simulink model "F103_0804_simulink_model"  (R2025b)
settings: Solver=FixedStepDiscrete  StartTime=0.0  StopTime=10.0  FixedStep=0.01  RelTol=1e-3  EnableMultiTasking=on
settings Model: Creator=Admin1  LastModifiedBy=Admin1
settings SolverCC: AutoInsertRateTranBlk=on
settings OptimizationCC: DefaultParameterBehavior=Inlined  UseDivisionForNetSlopeComputation=on  GainParamInheritBuiltInType=on  UseFloatMulNetSlope=on  InlineInvariantSignals=on  PassReuseOutputArgsAs=Individual arguments  ZeroExternalMemoryAtStartup=off  ZeroInternalMemoryAtStartup=off  NoFixptDivByZeroProtection=on  EfficientFloat2IntCast=on  LifeSpan=1  OptimizeBlockOrder=speed  DifferentSizesBufferReuse=on  EfficientTunableParamExpr=on
settings DebuggingCC: ParameterTunabilityLossMsg=error
settings HardwareCC: ProdBitPerPointer=32.0  ProdBitPerSizeT=32.0  ProdBitPerPtrDiffT=32.0  ProdLargestAtomicInteger=Long  ProdLargestAtomicFloat=Double  ProdWordSize=32.0  ProdLongLongMode=on  ProdHWDeviceType=ARM Compatible->STM32Processor
settings SFSimCC: SimCustomHeaderCode=bms_app.h  SimUserSources=bms_app.c  SimUserIncludeDirs=D:\FSAE_CHD\BMS\STM32_LTC68xx_BMS_Chang-an\F407_VET6_Test\Appl  MATLABDynamicMemAlloc=off
settings RTWCC: SystemTargetFile=ert.tlc  GenCodeOnly=on  TemplateMakefile=ert_default_tmf  CustomHeaderCode=bms_app.h  CustomInclude=D:\FSAE_CHD\BMS\STM32_LTC68xx_BMS_Chang-an\F407_VET6_Test\Appl  CustomSource=bms_app.c  Description=Embedded Coder
settings CodeAppCC: ForceParamTrailComments=on  IgnoreCustomStorageClasses=off  OperatorAnnotations=on  SimulinkDataObjDesc=on  SFDataObjDesc=on  CustomSymbolStrGlobalVar=rt$N$M  CustomSymbolStrType=$N$M  CustomSymbolStrFcn=$N$M$F  CustomSymbolStrMacro=$N$M  InsertBlockDesc=on
settings ERTTargetCC: ERTCustomFileTemplate=example_file_process.tlc  ERTFilePackagingFormat=CompactWithDataFile  TargetLangStandard=C99 (ISO)  IncludeMdlTerminateFcn=off  CombineSignalStateStructs=on  SupportAbsoluteTime=off  SupportComplex=off  SupportNonInlinedSFcns=on

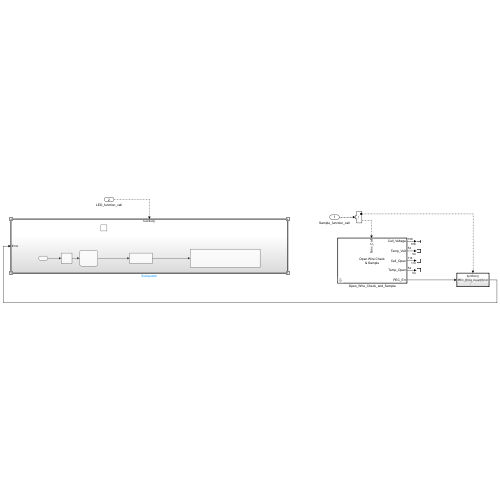
[thumbnail: Simulink's stored preview of the top-level diagram]
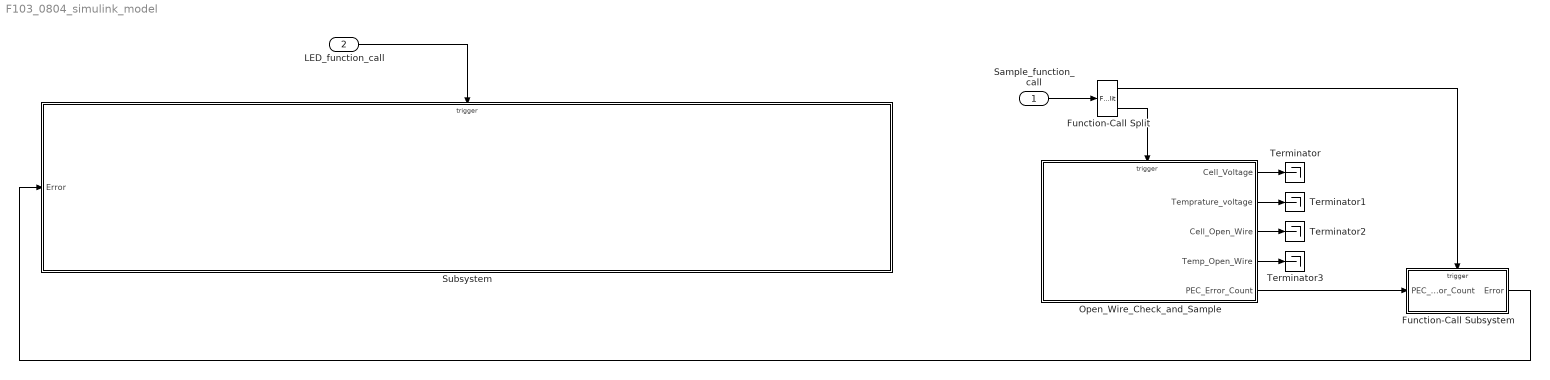
== system F103_0804_simulink_model ==
  Sample_function_call : Inport  SampleTime=0.01  OutputFunctionCall=on
  LED_function_call : Inport  Port=2  SampleTime=0.01  OutputFunctionCall=on
  Function-Call Split : FunctionCallSplit  IconShape=distinctive  NumOutputPorts=2  OutputPortLayout=default
  Function-Call Subsystem : Subsystem  TreatAsAtomicUnit=on
  Open_Wire_Check_and_Sample : Subsystem  TreatAsAtomicUnit=on
      mask DialogControl ParameterGroupVar Prompt: 参数
      mask Display:
      | disp('Open Wire Check\n& Sample');
      | port_label('input',1,'Func_Call');
      | port_label('output',1,'Cell_Voltage');
      | port_label('output',2,'Temp_Volt');
      | port_label('output',3,'Cell_Open');
      | port_label('output',4,'Temp_Open');
      | port_label('output',5,'PEC_Err');
  Subsystem : Subsystem
  Terminator{,1..3} (4 alike) : Terminator
  wires:
  Open_Wire_Check_and_Sample/1(Cell_Voltage) -> Terminator/1
  Open_Wire_Check_and_Sample/2(Temprature_voltage) -> Terminator1/1
  Open_Wire_Check_and_Sample/3(Cell_Open_Wire) -> Terminator2/1
  Open_Wire_Check_and_Sample/4(Temp_Open_Wire) -> Terminator3/1
  LED_function_call/1 -> Subsystem/Trigger
  Open_Wire_Check_and_Sample/5(PEC_Error_Count) -> Function-Call Subsystem/1(PEC_Error_Count)
  Sample_function_call/1 -> Function-Call Split/1
  Function-Call Split/2 -> Open_Wire_Check_and_Sample/Trigger
  Function-Call Split/1 -> Function-Call Subsystem/Trigger
  Function-Call Subsystem/1(Error) -> Subsystem/1(Error)

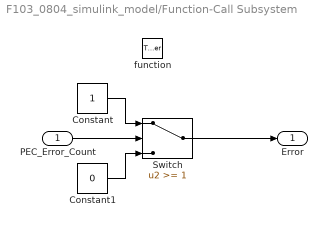
== system F103_0804_simulink_model/Function-Call Subsystem ==
  PEC_Error_Count : Inport
  function : TriggerPort  TriggerType=function-call  VariantControl=(inherit)  SampleTimeType=periodic  SampleTime=0.01
  Constant : Constant
  Constant1 : Constant  Value=0
  Switch : Switch  Threshold=1  SaturateOnIntegerOverflow=off  InputSameDT=off
  Error : Outport
  wires:
  PEC_Error_Count/1 -> Switch/2
  Constant/1 -> Switch/1
  Constant1/1 -> Switch/3
  Switch/1 -> Error/1

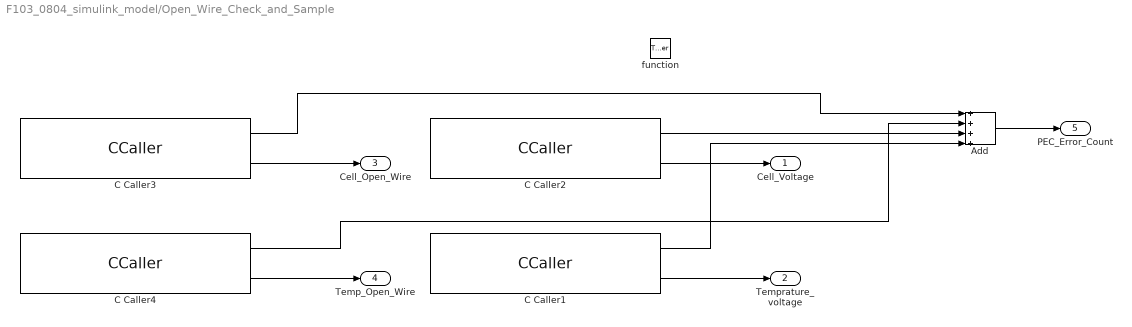
== system F103_0804_simulink_model/Open_Wire_Check_and_Sample ==
  function : TriggerPort  TriggerType=function-call  VariantControl=(inherit)  SampleTimeType=periodic  SampleTime=0.01
  Add : Sum  Inputs=++++
  C Caller1 : CCaller  Priority=3  FunctionName=Bms_SampleTemperature  PortSpecificationStruct="%)30     .    R ,   8    (     @         %    \"     (    !     0         %  0 \"0    $    _    07)G3F%M90  4&]R=$YA;64 4V-O<&4     26YD97@     5'EP90      4VEZ90      27-';&]B86P   X    P    !@    @    $          4    (     0    ,    !         !   P!O=70 #@   #     &    \"     0         !0    @    !     P    $         $  # &]U=  .    .     8    (    !          %    \"     $    &     0         0    !@   $]U='!U=   #@   #@    &    \"     8         !0    @    !     0    $         \"0    @               X    X    !@    @    $          4    (     0    4    !         !     %    =6EN=#@    .    ,     8    (    !          %    \"     $    !     0         0  $ ,0    X    P    !@    @    ) @        4    (     0    $    !          (  0      #@   #@    &    \"     0         !0    @    !    !0    $         $     4   !C;V1E<P    X    X    !@    @    $          4    (     0    4    !         !     %    8V]D97,    .    .     8    (    !          %    \"     $    &     0         0    !@   $]U='!U=   #@   #@    &    \"     8         !0    @    !     0    $         \"0    @           #P/PX    X    !@    @    $          4    (     0    8    !         !     &    =6EN=#$V   .    ,     8    (    !          %    \"     $    \"     0         0  ( -30   X    P    !@    @    ) @        4    (     0    $    !          (  0"
  C Caller2 : CCaller  Priority=2  FunctionName=Bms_SampleCellVoltage  PortSpecificationStruct="%)30     .    R ,   8    (     @         %    \"     (    !     0         %  0 \"0    $    _    07)G3F%M90  4&]R=$YA;64 4V-O<&4     26YD97@     5'EP90      4VEZ90      27-';&]B86P   X    P    !@    @    $          4    (     0    ,    !         !   P!O=70 #@   #     &    \"     0         !0    @    !     P    $         $  # &]U=  .    .     8    (    !          %    \"     $    &     0         0    !@   $]U='!U=   #@   #@    &    \"     8         !0    @    !     0    $         \"0    @               X    X    !@    @    $          4    (     0    4    !         !     %    =6EN=#@    .    ,     8    (    !          %    \"     $    !     0         0  $ ,0    X    P    !@    @    ) @        4    (     0    $    !          (  0      #@   #@    &    \"     0         !0    @    !    !0    $         $     4   !C;V1E<P    X    X    !@    @    $          4    (     0    4    !         !     %    8V]D97,    .    .     8    (    !          %    \"     $    &     0         0    !@   $]U='!U=   #@   #@    &    \"     8         !0    @    !     0    $         \"0    @           #P/PX    X    !@    @    $          4    (     0    8    !         !     &    =6EN=#$V   .    ,     8    (    !          %    \"     $    #     0         0  , ,3 X  X    P    !@    @    ) @        4    (     0    $    !          (  0"
  C Caller3 : CCaller  Priority=0  FunctionName=Bms_DetectCellOpenWire  PortSpecificationStruct="%)30     .    R ,   8    (     @         %    \"     (    !     0         %  0 \"0    $    _    07)G3F%M90  4&]R=$YA;64 4V-O<&4     26YD97@     5'EP90      4VEZ90      27-';&]B86P   X    P    !@    @    $          4    (     0    ,    !         !   P!O=70 #@   #     &    \"     0         !0    @    !     P    $         $  # &]U=  .    .     8    (    !          %    \"     $    &     0         0    !@   $]U='!U=   #@   #@    &    \"     8         !0    @    !     0    $         \"0    @               X    X    !@    @    $          4    (     0    4    !         !     %    =6EN=#@    .    ,     8    (    !          %    \"     $    !     0         0  $ ,0    X    P    !@    @    ) @        4    (     0    $    !          (  0      #@   #@    &    \"     0         !0    @    !    !0    $         $     4   !F;&%G<P    X    X    !@    @    $          4    (     0    4    !         !     %    9FQA9W,    .    .     8    (    !          %    \"     $    &     0         0    !@   $]U='!U=   #@   #@    &    \"     8         !0    @    !     0    $         \"0    @           #P/PX    X    !@    @    $          4    (     0    4    !         !     %    =6EN=#@    .    ,     8    (    !          %    \"     $    #     0         0  , ,3$T  X    P    !@    @    ) @        4    (     0    $    !          (  0"
  C Caller4 : CCaller  Priority=1  FunctionName=Bms_DetectTempOpenWire  PortSpecificationStruct="%)30     .    R ,   8    (     @         %    \"     (    !     0         %  0 \"0    $    _    07)G3F%M90  4&]R=$YA;64 4V-O<&4     26YD97@     5'EP90      4VEZ90      27-';&]B86P   X    P    !@    @    $          4    (     0    ,    !         !   P!O=70 #@   #     &    \"     0         !0    @    !     P    $         $  # &]U=  .    .     8    (    !          %    \"     $    &     0         0    !@   $]U='!U=   #@   #@    &    \"     8         !0    @    !     0    $         \"0    @               X    X    !@    @    $          4    (     0    4    !         !     %    =6EN=#@    .    ,     8    (    !          %    \"     $    !     0         0  $ ,0    X    P    !@    @    ) @        4    (     0    $    !          (  0      #@   #@    &    \"     0         !0    @    !    !0    $         $     4   !F;&%G<P    X    X    !@    @    $          4    (     0    4    !         !     %    9FQA9W,    .    .     8    (    !          %    \"     $    &     0         0    !@   $]U='!U=   #@   #@    &    \"     8         !0    @    !     0    $         \"0    @           #P/PX    X    !@    @    $          4    (     0    4    !         !     %    =6EN=#@    .    ,     8    (    !          %    \"     $    \"     0         0  ( -30   X    P    !@    @    ) @        4    (     0    $    !          (  0"
  Cell_Voltage : Outport
  Temprature_voltage : Outport  Port=2
  Cell_Open_Wire : Outport  Port=3
  Temp_Open_Wire : Outport  Port=4
  PEC_Error_Count : Outport  Port=5
  wires:
  C Caller2/2 -> Cell_Voltage/1
  C Caller1/2 -> Temprature_voltage/1
  C Caller3/2 -> Cell_Open_Wire/1
  C Caller4/2 -> Temp_Open_Wire/1
  C Caller3/1 -> Add/1
  C Caller4/1 -> Add/2
  C Caller2/1 -> Add/3
  C Caller1/1 -> Add/4
  Add/1 -> PEC_Error_Count/1

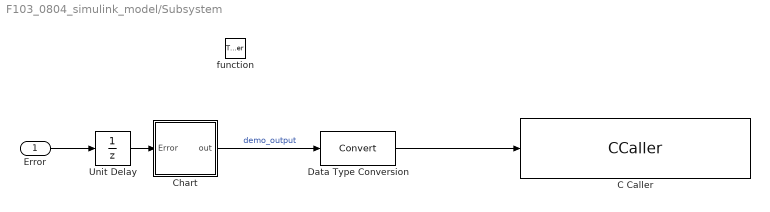
== system F103_0804_simulink_model/Subsystem ==
  Error : Inport
  function : TriggerPort  TriggerType=function-call  VariantControl=(inherit)  SampleTimeType=periodic  SampleTime=0.01
  C Caller : CCaller  FunctionName=Bms_LED_Control  PortSpecificationStruct="%)30     .    & (   8    (     @         %    \"     $    !     0         %  0 \"0    $    _    07)G3F%M90  4&]R=$YA;64 4V-O<&4     26YD97@     5'EP90      4VEZ90      27-';&]B86P   X    P    !@    @    $          4    (     0    (    !         !   @!O;@  #@   #     &    \"     0         !0    @    !     @    $         $  \" &]N   .    .     8    (    !          %    \"     $    %     0         0    !0   $EN<'5T    #@   #@    &    \"     8         !0    @    !     0    $         \"0    @               X    X    !@    @    $          4    (     0    4    !         !     %    =6EN=#@    .    ,     8    (    !          %    \"     $    !     0         0  $ ,0    X    P    !@    @    ) @        4    (     0    $    !          (  0"
  Chart : Stateflow chart  TreatAsAtomicUnit=on
  Data Type Conversion : DataTypeConversion  SaturateOnIntegerOverflow=off  RndMeth=Floor
  Unit Delay : UnitDelay  SampleTime=-1  HasFrameUpgradeWarning=on
  wires:
  Data Type Conversion/1 -> C Caller/1
  Chart/1(out) -> Data Type Conversion/1  "demo_output"
  Error/1 -> Unit Delay/1
  Unit Delay/1 -> Chart/1(Error)

== stateflow chart F103_0804_simulink_model/Subsystem/Chart ==
  state OFF
    en:
    out = 0;
  state ON
    en:
    out = 1;
  state Error_OFF
    en:
    out = 0;
  state Error_ON
    en:
    out = 1;
  (default) -> OFF
  OFF -> ON [order 1] : after(3,sec)
  ON -> OFF [order 1] : after(3,sec)
  OFF -> Error_OFF [order 2] : [Error == 1]
  ON -> Error_ON [order 2] : [Error == 1]
  Error_OFF -> Error_ON : after(0.1,sec)
  Error_ON -> Error_OFF : after(0.1,sec)
  data: out output uint8; Error input
